simulink model "voltmult"  (R2015a)
settings: Solver=ode23t  StartTime=0.0  StopTime=1.0  RelTol=1e-3
libraries: powerlib x15, powerlib_meascontrol x2
settings Model: Creator=asus  LastModifiedBy=asus

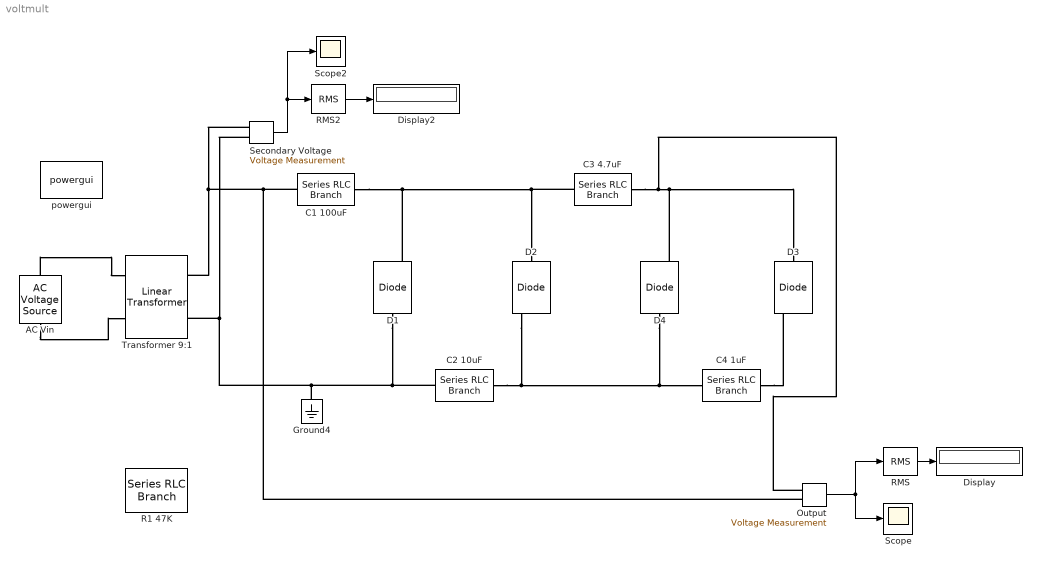
== system voltmult ==
  AC Vin : powerlib/Electrical Sources/AC Voltage Source  Amplitude=220*sqrt(2)  Phase=0  Frequency=60  SampleTime=0  Measurements=None
  C1 100uF : powerlib/Elements/Series RLC Branch  LConnTagsString=__new0  RConnTagsString=__new0  BranchType=C  Resistance=0  Inductance=0  SetiL0=off  InitialCurrent=0  Capacitance=100e-6  Setx0=off  InitialVoltage=0  Measurements=None
  C2 10uF : powerlib/Elements/Series RLC Branch  LConnTagsString=__new0  RConnTagsString=__new0  BranchType=C  Resistance=0  Inductance=0  SetiL0=off  InitialCurrent=0  Capacitance=10e-6  Setx0=off  InitialVoltage=0  Measurements=None
  C3 4.7uF : powerlib/Elements/Series RLC Branch  LConnTagsString=__new0  RConnTagsString=__new0  BranchType=C  Resistance=0  Inductance=0  SetiL0=off  InitialCurrent=0  Capacitance=4.7e-6  Setx0=off  InitialVoltage=0  Measurements=None
  C4 1uF : powerlib/Elements/Series RLC Branch  LConnTagsString=__new0  RConnTagsString=__new0  BranchType=C  Resistance=0  Inductance=0  SetiL0=off  InitialCurrent=0  Capacitance=1e-6  Setx0=off  InitialVoltage=0  Measurements=None
  D{1..4} (4 alike) : powerlib/Power Electronics/Diode  Ron=0.001  Lon=0  Vf=0.8  IC=0  UseSnubber=off  Rs=0  Cs=0  Measurements=on
  Display : Display
  Display2 : Display
  Ground4 : powerlib/Elements/Ground  LConnTagsString=a
  Output : powerlib/Measurements/Voltage Measurement  PhasorSimulation=off  OutputType=Complex  PSBequivalent=0
  R1 47K : powerlib/Elements/Series RLC Branch  LConnTagsString=__new0  RConnTagsString=__new0  BranchType=R  Resistance=47000  Inductance=0  SetiL0=off  InitialCurrent=0  Capacitance=100e-6  Setx0=off  InitialVoltage=0  Measurements=None
  RMS : powerlib_meascontrol/Measurements/RMS  TrueRMS=on  Freq=60  RMSInit=120  Ts=0
  RMS2 : powerlib_meascontrol/Measurements/RMS  TrueRMS=on  Freq=60  RMSInit=120  Ts=0
  Scope : Scope
  Scope2 : Scope
  Secondary Voltage : powerlib/Measurements/Voltage Measurement  PhasorSimulation=off  OutputType=Complex  PSBequivalent=0
  Transformer 9:1 : powerlib/Elements/Linear Transformer  UNITS=SI  NominalPower=[ 250e6 60 ]  winding1=[220 0 0]  winding2=[220/9 0 0]  ThreeWindings=off  winding3=[12 0 0]  RmLm=[inf inf]  Measurements=None  DataType=on
  powergui : powerlib/powergui  Priority=1  SimulationMode=Discrete  SolverType=Tustin/Backward Euler (TBE)  SampleTime=10e-6  frequency=60  SPID=off  DisableSnubberDevices=off  DisableRonSwitches=off  DisableVfSwitches=off  SwTol=0  DisplayEquations=off  Interpol=on  methode=off  Ts=100  FunctionMessages=off  echomessages=off  HookPort=off  EnableUseOfTLC=off  x0status=blocks  frequencyindice=60  Pbase=100e6  ErrMax=1e-4  Iterations=50  UnitsV=kV  UnitsW=MW  buscounter=0  RestoreLinks=warning  ResistiveCurrentMeasurement=off  Frange=[0:2:500]  Ylog=off  Xlog=on  ShowGrid=off  save=off  variable=ZData  structure=0  ZoomFFT=off  StartTime=0.0  cycles=1  DisplayStyle=1  fundamental=60  FreqAxis=off  MaxFrequency=1000  frequencyindicesteady=1  RmsSteady=1  display=off
  wires:
  Output/1 -> RMS/1, Scope/1
  RMS/1 -> Display/1
  Secondary Voltage/1 -> Scope2/1, RMS2/1
  RMS2/1 -> Display2/1
  connections:
  AC Vin/RConn1 -- Transformer 9:1/LConn1
  AC Vin/LConn1 -- Transformer 9:1/LConn2
  Transformer 9:1/RConn1 -- Output/LConn2 -- C1 100uF/RConn1 -- Secondary Voltage/LConn1
  Secondary Voltage/LConn2 -- C2 10uF/RConn1 -- D1/LConn1 -- Ground4/LConn1 -- Transformer 9:1/RConn2
  D4/RConn1 -- Output/LConn1 -- C3 4.7uF/LConn1 -- D3/LConn1
  C1 100uF/LConn1 -- D1/RConn1 -- C3 4.7uF/RConn1 -- D2/LConn1
  C4 1uF/LConn1 -- D3/RConn1
  D4/LConn1 -- C2 10uF/LConn1 -- D2/RConn1 -- C4 1uF/RConn1
